simulink library "pathPositionNumerical_ul"  (R2018b)
settings: Solver=VariableStepAuto  StartTime=0.0  StopTime=10.0  RelTol=1e-3
settings Model: Creator=mcobb  LastModifiedBy=mitch
settings DebuggingCC: LibraryContextMissingDiagnostic=none
settings SFSimCC: SimUseLocalCustomCode=off
settings RTWCC: RTWUseLocalCustomCode=off

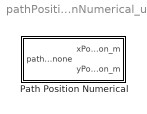
== system pathPositionNumerical_ul ==
  Path Position Numerical : Subsystem  mask{brkpts=0, xVals=0, yVals=0}
      mask prompts: brkpts "Breakpoints"; xVals "X Values"; yVals "Y Values"

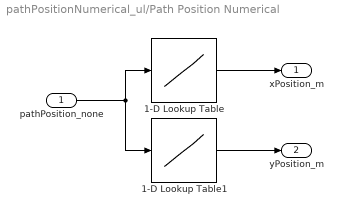
== system pathPositionNumerical_ul/Path Position Numerical ==
  pathPosition_none : Inport
  1-D Lookup Table : Lookup_n-D  NumberOfTableDimensions=1  BreakpointsForDimension1=brkpts  Table=xVals  InternalRulePriority=Speed  RndMeth=Simplest  InputSameDT=on
  1-D Lookup Table1 : Lookup_n-D  NumberOfTableDimensions=1  BreakpointsForDimension1=brkpts  Table=yVals  InternalRulePriority=Speed  RndMeth=Simplest  InputSameDT=on
  xPosition_m : Outport
  yPosition_m : Outport  Port=2
  wires:
  1-D Lookup Table/1 -> xPosition_m/1
  1-D Lookup Table1/1 -> yPosition_m/1
  pathPosition_none/1 -> 1-D Lookup Table1/1, 1-D Lookup Table/1
